simulink model "Asenkron_Motorun_Yumusak_Baslatilmasi"  (R2024b)
settings: Solver=VariableStepAuto  StartTime=0.0  StopTime=2.0  RelTol=1e-3
undefined symbols (not defined in the file): D1, lagging, pulse
libraries: spsThyristorLib x6, spsRMSLib x4, spsACVoltageSourceLib x3, spsThreePhaseVIMeasurementLib x2, spsAsynchronousMachineSIUnitsLib x1, spsGroundLib x1, spsPLL3phLib x1, spsPulseGeneratorThyristor6PulseLib x1, spspowerguiLib x1
settings Model: Creator=serca  LastModifiedBy=jraza
settings RTWCC: GPUComputeCapability=3.5

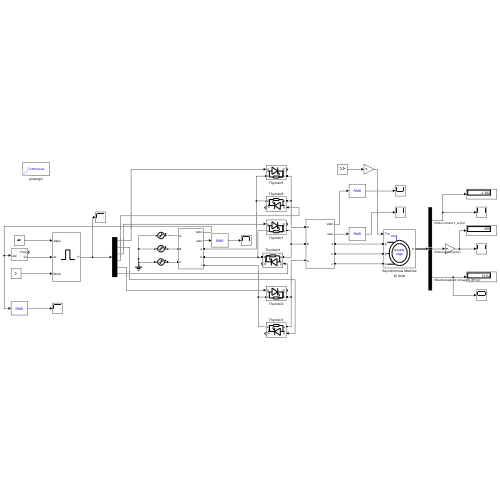
[thumbnail: Simulink's stored preview of the top-level diagram]
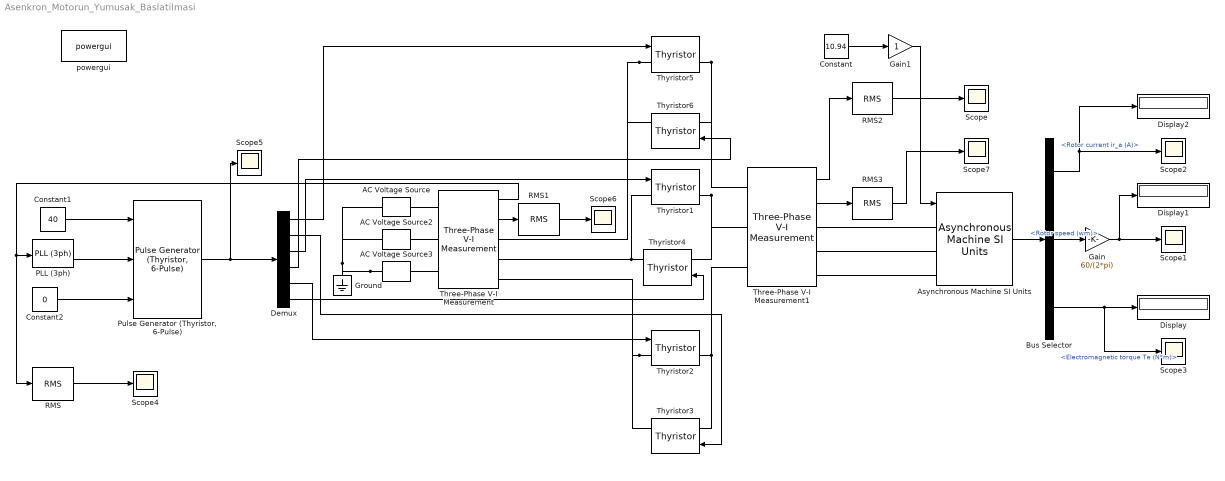
== system Asenkron_Motorun_Yumusak_Baslatilmasi ==
  AC Voltage Source : spsACVoltageSourceLib/AC Voltage Source  Amplitude=400  Phase=0  Frequency=50  SampleTime=0  Measurements=None  BusType=swing  Pref=10e3  Qref=0  Qmin=-inf  Qmax=+inf
  AC Voltage Source2 : spsACVoltageSourceLib/AC Voltage Source  Amplitude=400  Phase=-120  Frequency=50  SampleTime=0  Measurements=None  BusType=swing  Pref=10e3  Qref=0  Qmin=-inf  Qmax=+inf
  AC Voltage Source3 : spsACVoltageSourceLib/AC Voltage Source  Amplitude=400  Phase=120  Frequency=50  SampleTime=0  Measurements=None  BusType=swing  Pref=10e3  Qref=0  Qmin=-inf  Qmax=+inf
  Asynchronous Machine SI Units : spsAsynchronousMachineSIUnitsLib/Asynchronous Machine SI Units  RotorType=Double squirrel-cage  PresetModel=No  MechanicalLoad=Torque Tm  ShowDetailedParameters=on  ReferenceFrame=Rotor  Units=SI  MeasurementBus=off  NominalParameters=[1100 400 50]  VoltageRatio=1  Stator=[4.201 0.02986]  Rotor=[1.395 0.005839]  Cage1=[9.56 0.0681]  Cage2=[9.589 0.02986]  Lm=0.564  Mechanical=[0.05 0.00334 3]  PolePairs=3  InitialConditions=[0.04 0 0 0 0 0 -120 120]  SimulateSaturation=off  Saturation=[14.03593122, 27.81365428, 53.79336849, 72.68890987, 97.98006896, 148.6815601, 215.7428561, 302.9841135, 428.7778367 ; 230, 322, 414, 460, 506, 552, 598, 644, 690]  LoadFlowParameters=1492000  TsPowergui=0  TsBlock=-1  IterativeModel=Trapezoidal non iterative  IterativeDiscreteModel=Trapezoidal non iterative  Pmec=0
  Bus Selector : BusSelector  OutputSignals=Rotor measurements.Rotor current ir_a (A),Mechanical.Rotor speed (wm),Mechanical.Electromagnetic torque Te (N*m)
  Constant : Constant  Value=10.94
  Constant1 : Constant  Value=40
  Constant2 : Constant  Value=0
  Demux : Demux  Outputs=6
  Display : Display
  Display1 : Display
  Display2 : Display
  Gain : Gain  Gain=60/(2*pi)
  Gain1 : Gain
  Ground : spsGroundLib/Ground  LConnTagsString=a
  PLL (3ph) : spsPLL3phLib/PLL (3ph)  Fmin=45  Par_Init=[0, 60]  ParK=[180, 3200, 1]  TcD=1e-4  MaxRateChangeFreq=12  FilterCutOffFreq=25  Ts=0  AGC=on
  "Pulse Generator (Thyristor, 6-Pulse)" : spsPulseGeneratorThyristor6PulseLib/Pulse Generator (Thyristor, 6-Pulse)  GenType=6-pulse  Delta=D1 (lagging)  pwidth=50  Double_Pulse=on  Ts=0
  RMS{,1..3} (4 alike) : spsRMSLib/RMS  TrueRMS=on  Freq=60  RMSInit=120  Ts=0
  Scope{,1..7} (8 alike) : Scope
  Three-Phase V-I Measurement : spsThreePhaseVIMeasurementLib/Three-Phase V-I Measurement  VoltageMeasurement=phase-to-ground  SetLabelV=off  LabelV=Vabc  Vpu=off  VpuLL=off  CurrentMeasurement=yes  SetLabelI=off  LabelI=Iabc  Ipu=off  Pbase=100e6  Vbase=500e3  OutputType=Complex  PhasorSimulation=off  PSBequivalent=0
  Three-Phase V-I Measurement1 : spsThreePhaseVIMeasurementLib/Three-Phase V-I Measurement  VoltageMeasurement=phase-to-ground  SetLabelV=off  LabelV=Vabc  Vpu=off  VpuLL=off  CurrentMeasurement=yes  SetLabelI=off  LabelI=Iabc  Ipu=off  Pbase=100e6  Vbase=500e3  OutputType=Complex  PhasorSimulation=off  PSBequivalent=0
  Thyristor{1..6} (6 alike) : spsThyristorLib/Thyristor  Ron=0.001  Lon=0  Vf=0.8  IC=0  Rs=500  Cs=250e-9  Measurements=on
  powergui : spspowerguiLib/powergui  Priority=1  SimulationMode=Continuous  SampleTime=50e-6  frequency=60  Iterations=50  frequencyindice=50  Pbase=100e6  ErrMax=1e-4  UnitsV=kV  UnitsW=MW  buscounter=0  FunctionMessages=off  echomessages=off  EnableUseOfTLC=off  CurrentSourceSwitches=off  DisableSnubberDevices=off  DisableRonSwitches=off  DisableVfSwitches=off  DisplayEquations=off  AutomaticDiscreteSolvers=off  SolverType=Tustin/Backward Euler (TBE)  Interpol=off  ExternalGateDelay=off  methode=off  Ts=100  x0status=blocks  SPID=on  SwTol=0  HookPort=off  NonlinearTolerance=1e-4  nMaxIteration=100  ContinueOnMaxIteration=off  RestoreLinks=warning  ResistiveCurrentMeasurement=off  Frange=[0:2:500]  Ylog=off  Xlog=on  ShowGrid=off  save=off  variable=ZData  structure=0  ZoomFFT=off  StartTime=0.0  cycles=1  DisplayStyle=1  fundamental=60  FreqAxis=off  MaxFrequency=1000  frequencyindicesteady=1  RmsSteady=1  display=off
  wires:
  Constant1/1 -> "Pulse Generator (Thyristor, 6-Pulse)"/1
  Demux/6 -> Thyristor4/1
  Three-Phase V-I Measurement1/2 -> RMS3/1
  RMS1/1 -> Scope6/1
  Gain/1 -> Display1/1, Scope1/1
  RMS3/1 -> Scope7/1
  RMS/1 -> Scope4/1
  Three-Phase V-I Measurement/2 -> RMS1/1
  Three-Phase V-I Measurement1/1 -> RMS2/1
  Demux/3 -> Thyristor1/1
  RMS2/1 -> Scope/1
  Constant2/1 -> "Pulse Generator (Thyristor, 6-Pulse)"/3
  Demux/4 -> Thyristor6/1
  Gain1/1 -> Asynchronous Machine SI Units/1
  Demux/1 -> Thyristor5/1
  Demux/5 -> Thyristor2/1
  Demux/2 -> Thyristor3/1
  "Pulse Generator (Thyristor, 6-Pulse)"/1 -> Demux/1, Scope5/1
  PLL (3ph)/2 -> "Pulse Generator (Thyristor, 6-Pulse)"/2
  Constant/1 -> Gain1/1
  Bus Selector/1 -> Display2/1, Scope2/1  "<Rotor current ir_a (A)>"
  Bus Selector/2 -> Gain/1  "<Rotor speed (wm)>"
  Bus Selector/3 -> Display/1, Scope3/1  "<Electromagnetic torque Te (N*m)>"
  Three-Phase V-I Measurement/1 -> RMS/1, PLL (3ph)/1
  Asynchronous Machine SI Units/1 -> Bus Selector/1
  connections:
  Thyristor2/LConn1 -- Three-Phase V-I Measurement/RConn3 -- Thyristor3/RConn1
  Thyristor2/RConn1 -- Thyristor3/LConn1 -- Three-Phase V-I Measurement1/LConn3
  Thyristor5/RConn1 -- Thyristor6/LConn1 -- Three-Phase V-I Measurement1/LConn1
  AC Voltage Source3/LConn1 -- AC Voltage Source/LConn1 -- AC Voltage Source2/LConn1 -- Ground/LConn1
  Thyristor5/LConn1 -- Thyristor6/RConn1 -- Three-Phase V-I Measurement/RConn1
  Thyristor1/RConn1 -- Thyristor4/LConn1 -- Three-Phase V-I Measurement1/LConn2
  Thyristor4/RConn1 -- Thyristor1/LConn1 -- Three-Phase V-I Measurement/RConn2
  AC Voltage Source3/RConn1 -- Three-Phase V-I Measurement/LConn3
  AC Voltage Source/RConn1 -- Three-Phase V-I Measurement/LConn1
  Three-Phase V-I Measurement1/RConn3 -- Asynchronous Machine SI Units/LConn3
  Three-Phase V-I Measurement1/RConn2 -- Asynchronous Machine SI Units/LConn2
  AC Voltage Source2/RConn1 -- Three-Phase V-I Measurement/LConn2
  Three-Phase V-I Measurement1/RConn1 -- Asynchronous Machine SI Units/LConn1
